simulink model "FirstCode_ControlHarness"  (R2014b)
settings: Solver=FixedStepDiscrete  StartTime=0.0  StopTime=5  RelTol=1e-3
PostLoadFcn:
  | c2000demoscallback(1)
model workspace: external: MAT-File (data not in the file)
undefined symbols (not defined in the file or in its folder): canChannel
libraries: canlib x3, canmsglib x2, realtime_pacer_lib x1
settings Model: Creator=The MathWorks Inc.  LastModifiedBy=Nathan
settings DataIOCC: SignalLoggingSaveFormat=ModelDataLogs  SaveOutput=off  SaveTime=off
settings OptimizationCC: ExpressionDepthLimit=2147483647  InitFltsAndDblsToZero=on  OptimizeModelRefInitCode=on  LifeSpan=Inf  MaxStackSize=64
settings DebuggingCC: UnderspecifiedInitializationDetection=Classic  MergeDetectMultiDrivingBlocksExec=none  SignalResolutionControl=TryResolveAllWithWarning  SolverPrmCheckMsg=none  InheritedTsInSrcMsg=none  MultiTaskDSMMsg=warning  MultiTaskCondExecSysMsg=none  FcnCallInpInsideContextMsg=UseLocalSettings  StateNameClashWarn=warning
settings HardwareCC: ProdBitPerChar=16  ProdBitPerInt=16  ProdBitPerPointer=16  ProdLargestAtomicInteger=Integer  ProdIntDivRoundTo=Zero  ProdEndianess=LittleEndian  ProdWordSize=16  ProdHWDeviceType=Texas Instruments->C2000  TargetBitPerChar=16  TargetBitPerInt=16  TargetBitPerPointer=16  TargetLargestAtomicInteger=Integer  TargetIntDivRoundTo=Zero  TargetEndianess=LittleEndian  TargetWordSize=16  TargetHWDeviceType=Texas Instruments->C2000
settings RTWCC: SystemTargetFile=ert.tlc  TemplateMakefile=ert_default_tmf  PostCodeGenCommand=; ;codertarget.postCodeGenHookCommand(h)  Description=Embedded Coder  GenerateReport=on  ProcessScript=ert_make_rtw_hook  Toolchain=Texas Instruments Code Composer Studio v5 (C2000)  BuildConfiguration=Faster Runs  IncludeHyperlinkInReport=on  PortableWordSizes=on  CodeExecutionProfiling=on  CodeProfilingInstrumentation=on
settings CodeAppCC: IgnoreCustomStorageClasses=off  CustomSymbolStrType=$N$R$M  InternalIdentifier=Classic

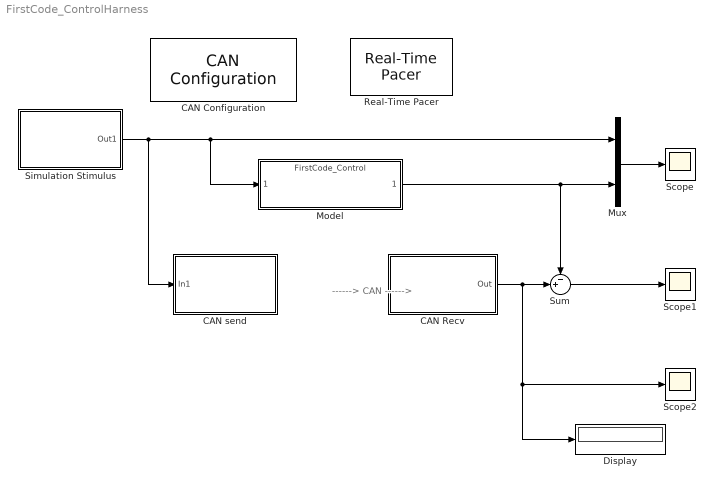
== system FirstCode_ControlHarness ==
  note: ------> CAN ------>
  CAN Configuration : canlib/CAN Configuration  BlockHandle=84.0184  DeviceMenu=Kvaser Eagle 1 (Channel 1)  Device=Kvaser Eagle 1 (Channel 1)  ObjConstructor=canChannel('Kvaser', 'Eagle 1', 1)  BusSpeed=500000  EnableBitParameters=off  SJW=1  TSEG1=4  TSEG2=3  NSamples=1  AckMode=Normal
  CAN Recv : Subsystem
  CAN send : Subsystem
  Display : Display
  Model : ModelReference  ModelNameDialog=FirstCode_Control.slx  SimulationMode=Normal  ModelReferenceVersion=1.85  CopyOfModelName=FirstCode_Control.slx  DefaultDataLogging=on
  Mux : Mux  Inputs=2
  Real-Time Pacer : realtime_pacer_lib/Real-Time Pacer  simTimePerRealTime=1
  Scope : Scope
  Scope1 : Scope
  Scope2 : Scope
      settings: TimeRange=10  SaveName=ScopeData2
  Simulation Stimulus : Subsystem
  Sum : Sum  Inputs=-+|
  wires:
  Simulation Stimulus/1(Out1) -> CAN send/1(In1), Model/1, Mux/1
  Mux/1 -> Scope/1
  CAN Recv/1(Out) -> Display/1, Scope2/1, Sum/2
  Sum/1 -> Scope1/1
  Model/1 -> Sum/1, Mux/2

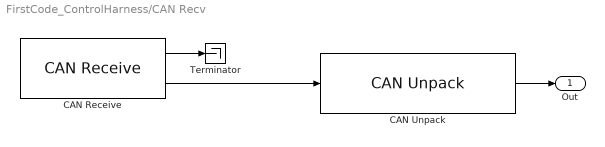
== system FirstCode_ControlHarness/CAN Recv ==
  CAN Receive : canlib/CAN Receive  BlockHandle=86.0007  DeviceMenu=Kvaser Eagle 1 (Channel 1)  Device=Kvaser Eagle 1 (Channel 1)  ObjConstructor=canChannel('Kvaser', 'Eagle 1', 1)  EnableStandardIDsFilter=off  StandardIDs=1  EnableExtendedIDsFilter=off  ExtendedIDs=0  SampleTime=.01  MsgsPerTimestep=all  StdIDsCombo=Allow only  ExtIDsCombo=Block all  InternalFilterUpdateStatus=on
  CAN Unpack : canmsglib/CAN Unpack  MsgList=(none)  MsgName=LED_Status  MsgIDType=Standard (11-bit identifier)  MsgIdentifier=1  MsgLength=2  SignalInfo=LED$0$16$1$1$1$0$1$0$-Inf$Inf$#  NSignals=1  IDPort=off  TimestampPort=off  ErrorPort=off  RemotePort=off  LengthPort=off  StatusPort=off  StartBits=str2num('[int32(0)]')  SignalSizes=str2num('[int32(16)]')  ByteOrders=str2num('[int32(1)]')  DataTypes=str2num('[int32(1)]')  MultiplexTypes=str2num('[int32(1)]')  MultiplexValues=str2num('[double(0)]')  Factors=str2num('[double(1)]')  Offsets=str2num('[double(0)]')  Minimums=str2num('[double(-Inf)]')  Maximums=str2num('[double(Inf)]')
  Terminator : Terminator
  Out : Outport
  wires:
  CAN Receive/1 -> Terminator/1
  CAN Receive/2 -> CAN Unpack/1
  CAN Unpack/1 -> Out/1

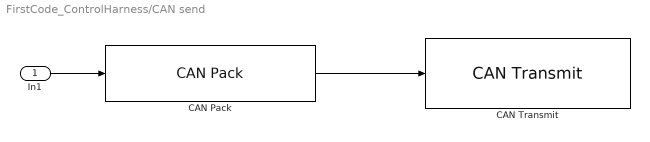
== system FirstCode_ControlHarness/CAN send ==
  In1 : Inport  OutDataTypeStr=int16
  CAN Pack : canmsglib/CAN Pack  MsgList=(none)  MsgName=Button_Press  MsgIDType=Standard (11-bit identifier)  MsgIdentifier=2  MsgLength=2  SignalInfo=Button$0$16$1$1$1$0$1$0$-Inf$Inf$#  NSignals=1  StartBits=str2num('[int32(0)]')  SignalSizes=str2num('[int32(16)]')  ByteOrders=str2num('[int32(1)]')  DataTypes=str2num('[int32(1)]')  MultiplexTypes=str2num('[int32(1)]')  MultiplexValues=str2num('[double(0)]')  Factors=str2num('[double(1)]')  Offsets=str2num('[double(0)]')  Minimums=str2num('[double(-Inf)]')  Maximums=str2num('[double(Inf)]')  Remote=off
      settings: DataFormat=manually specified signals
  CAN Transmit : canlib/CAN Transmit  BlockHandle=96.0007  DeviceMenu=Kvaser Eagle 1 (Channel 1)  Device=Kvaser Eagle 1 (Channel 1)  ObjConstructor=canChannel('Kvaser', 'Eagle 1', 1)  EnablePeriodicTransmit=on  MessagePeriod=.01
  wires:
  In1/1 -> CAN Pack/1
  CAN Pack/1 -> CAN Transmit/1

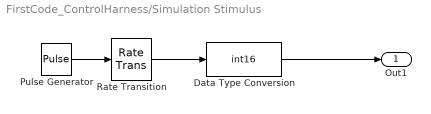
== system FirstCode_ControlHarness/Simulation Stimulus ==
  Data Type Conversion : DataTypeConversion  OutDataTypeStr=int16  RndMeth=Nearest
  Pulse Generator : DiscretePulseGenerator  PulseType=Time based  Amplitude=5  PulseWidth=50
  Rate Transition : RateTransition  OutPortSampleTime=0.01
  Out1 : Outport  OutDataTypeStr=int16
  wires:
  Pulse Generator/1 -> Rate Transition/1
  Rate Transition/1 -> Data Type Conversion/1
  Data Type Conversion/1 -> Out1/1
